simulink model "Microgrid"  (R2022b)
settings: Solver=ode45  StartTime=0.0  StopTime=0.5  RelTol=1e-3  EnableMultiTasking=on
model workspace (MAT data in the model file):
  AFPV = 1
  AFW = 1
  DG = 1
  pvc = 1
  wf1 = 1
undefined symbols (not defined in the file): BMSS1, D1, Delta, Ion, Lithium, R
libraries: spsDiodeLib x10, spsVoltageMeasurementLib x8, spsThreePhaseVIMeasurementLib x7, spsSeriesRLCBranchLib x7, fuzblock x6, spsMosfetLib x3, powerlib_extras x3, spsBreakerLib x2, spsThreePhaseParallelRLCLoadLib x2, spsThreePhaseBreakerLib x2, spsPWMGenerator2LevelLib x2, spsBatteryLib x1
(part 2 of 2)

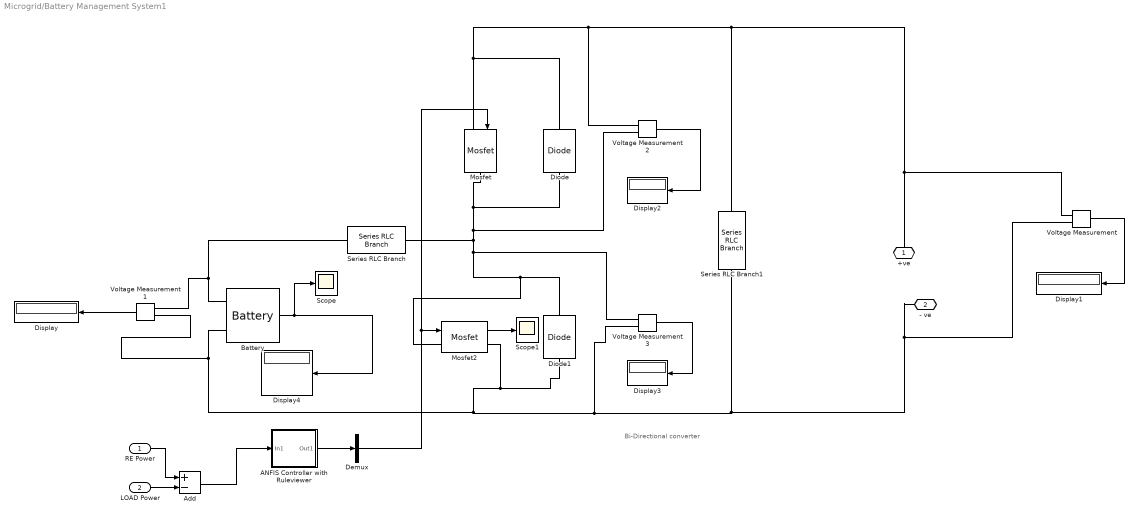
== system Microgrid/Battery Management System1 ==
  note: Bi-Directional converter
  RE Power : Inport
  LOAD Power : Inport  Port=2
  ANFIS Controller with Ruleviewer : Subsystem  AncestorBlock=|  mask(Fuzzy Inference System){fismatrix=[BMSS1], Ts=0.01}
      | fuzblock/Fuzzy Logic 
      | Controller 
      | with Ruleviewer
      mask prompts: fismatrix "fuzzy:dialogs:flcWithRuleViewerMaskPrompt_paramFIS"; Ts "fuzzy:dialogs:flcWithRuleViewerMaskPrompt_paramRate"
      mask help: fuzzy:dialogs:flcWithRuleViewerMask_description
      mask init:
      | fuzzy.internal.utility.errorIfType2FIS(fismatrix)
      settings: LibrarySourceBlock=|
      | fuzblock/Fuzzy Logic
      | Controller
      | with Ruleviewer
      mask Help: helpview(fullfile(docroot,'toolbox','fuzzy','fuzzy.map'), 'fuzviewerblock');
      mask DialogControl DescGroupVar Prompt: Fuzzy Inference System
      mask DialogControl fismatrix Prompt: FIS structure:
      mask DialogControl Ts Prompt: Refresh rate (s):
      mask Display: plot(0, -0.3, 6, -0.3, 0, 1.2, 6, 1.2, [0 6], [0 0], [1 2 3],[0 1 0],[2 3 4],[0 1 0],[3 4 5],[0 1 0])
  Add : Sum  Inputs=+-
  Battery : spsBatteryLib/Battery  BatType=Lithium-Ion  ShowTempParam=off  ThermalPreset=no  ShowAgeParam=off  NomV=200  NomQ=50  SOC=50  Batt_Tr=0.1  PresetModel=on  MaxQ=50  MinV=150  FullV=232.7974  Dis_rate=21.7391  R=0.04  Normal_OP=45.2174  expZone="[216.0772      2.456522]"  current=[5 10 15]  Units=Time  Tci=20  NomT=20  T2=-30  MaxQ2=4.8  FullV2=7.1  Normal_OP2=5.655  expZone2="[6.58           1]"  Rca=0.6  ti=2000  Dp=0  Neq0=0  Tsim=1e6  Ta1=25  Qeol=5.4*0.9  Reol=0.013333*1.2  Char_age=[2.3478, 3]  Dis_age=[2.3478, 10]  N1=1500  N2=10500  N3=1000  N4=1400  Ta2=45  N5=950
      settings: LibrarySourceBlock=electricdrivelib/Extra Sources/Battery
  Demux : Demux  Outputs=1
  Diode : spsDiodeLib/Diode  Ron=0.001  Lon=0  Vf=0.8  IC=0  UseSnubber=0  Rs=500  Cs=250e-9  Measurements=off
  Diode1 : spsDiodeLib/Diode  Ron=0.001  Lon=0  Vf=0.8  IC=0  UseSnubber=0  Rs=500  Cs=250e-9  Measurements=off
  Display{,1..4} (5 alike) : Display
  Mosfet : spsMosfetLib/Mosfet  Ron=0.1  Lon=0  Rd=0.01  Vfd=0  IC=0  Rs=1e5  Cs=inf  Measurements=off
  Mosfet2 : spsMosfetLib/Mosfet  Ron=0.1  Lon=0  Rd=0.01  Vfd=0  IC=0  Rs=1e5  Cs=inf  Measurements=on
  Scope : Scope
  Scope1 : Scope
  Series RLC Branch : spsSeriesRLCBranchLib/Series RLC Branch  LConnTagsString=__new0  RConnTagsString=__new0  BranchType=L  Resistance=1  Inductance=1e-3  SetiL0=off  InitialCurrent=0  Capacitance=1e-6  Setx0=off  InitialVoltage=0  Measurements=None
  Series RLC Branch1 : spsSeriesRLCBranchLib/Series RLC Branch  LConnTagsString=__new0  RConnTagsString=__new0  BranchType=RC  Resistance=1  Inductance=1e-3  SetiL0=off  InitialCurrent=0  Capacitance=1e-6  Setx0=off  InitialVoltage=0  Measurements=None
  Voltage Measurement{,1..3} (4 alike) : spsVoltageMeasurementLib/Voltage Measurement  PhasorSimulation=off  OutputType=Complex  PSBequivalent=0
  +ve : PMIOPort  Side=Right
  - ve : PMIOPort  Port=2  Side=Right
  wires:
  Voltage Measurement3/1 -> Display3/1
  Voltage Measurement2/1 -> Display2/1
  Voltage Measurement1/1 -> Display/1
  Voltage Measurement/1 -> Display1/1
  Battery/1 -> Scope/1, Display4/1
  ANFIS Controller with Ruleviewer/1(Out1) -> Demux/1
  Demux/1 -> Mosfet/1, Mosfet2/1
  Add/1 -> ANFIS Controller with Ruleviewer/1(In1)
  RE Power/1 -> Add/1
  LOAD Power/1 -> Add/2
  Mosfet2/1 -> Scope1/1
  connections:
  Mosfet/RConn1 -- Diode/LConn1 -- Voltage Measurement2/LConn2 -- Series RLC Branch/RConn1 -- Voltage Measurement3/LConn1 -- Mosfet2/LConn1 -- Diode1/RConn1
  Voltage Measurement1/LConn1 -- Series RLC Branch/LConn1 -- Battery/LConn1
  Mosfet/LConn1 -- Diode/RConn1 -- Voltage Measurement2/LConn1 -- Series RLC Branch1/LConn1 -- Voltage Measurement/LConn1 -- +ve/RConn1
  Diode1/LConn1 -- Mosfet2/RConn1 -- Battery/LConn2 -- Voltage Measurement1/LConn2 -- Voltage Measurement3/LConn2 -- Series RLC Branch1/RConn1 -- Voltage Measurement/LConn2 -- - ve/RConn1

== system Microgrid/Fuzzy Logic Controller with Ruleviewer ==
  In1 : Inport
  Fuzzy Logic Controller : fuzblock/Fuzzy Logic  Controller  FIS='tipper.fis'  OutputSampleNumber=101  DataType=double  FuzzifiedInputs=off  RuleFiringStrengths=off  RuleOutputs=off  AggregatedOutputs=off  SimulateUsing=Interpreted execution  OutOfRangeInputValueMessage=warning  NoRuleFiredMessage=warning  EmptyOutputFuzzySetMessage=warning
  Scope3 : Scope
  Zero-Order Hold : ZeroOrderHold  SampleTime=Ts
  Out1 : Outport  InitialOutput=0  VectorParamsAs1DForOutWhenUnconnected=off
  wires:
  In1/1 -> Fuzzy Logic Controller/1, Zero-Order Hold/1
  Fuzzy Logic Controller/1 -> Out1/1
  Zero-Order Hold/1 -> Scope3/1

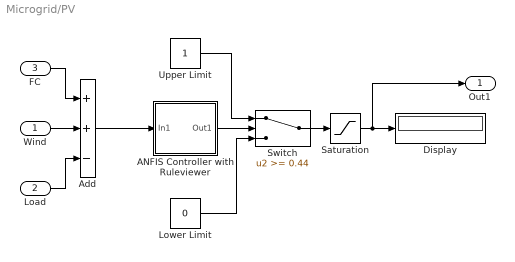
== system Microgrid/PV ==
  Wind : Inport
  Load : Inport  Port=2
  FC : Inport  Port=3
  ANFIS Controller with Ruleviewer : Subsystem  AncestorBlock=|  mask(Fuzzy Inference System){fismatrix=[pvc], Ts=0.01}
      | fuzblock/Fuzzy Logic 
      | Controller 
      | with Ruleviewer
      mask prompts: fismatrix "fuzzy:dialogs:flcWithRuleViewerMaskPrompt_paramFIS"; Ts "fuzzy:dialogs:flcWithRuleViewerMaskPrompt_paramRate"
      mask help: fuzzy:dialogs:flcWithRuleViewerMask_description
      mask init:
      | fuzzy.internal.utility.errorIfType2FIS(fismatrix)
      settings: LibrarySourceBlock=|
      | fuzblock/Fuzzy Logic
      | Controller
      | with Ruleviewer
      mask Help: helpview(fullfile(docroot,'toolbox','fuzzy','fuzzy.map'), 'fuzviewerblock');
      mask DialogControl DescGroupVar Prompt: Fuzzy Inference System
      mask DialogControl fismatrix Prompt: FIS structure:
      mask DialogControl Ts Prompt: Refresh rate (s):
      mask Display: plot(0, -0.3, 6, -0.3, 0, 1.2, 6, 1.2, [0 6], [0 0], [1 2 3],[0 1 0],[2 3 4],[0 1 0],[3 4 5],[0 1 0])
  Add : Sum  Inputs=++-
  Display : Display
  Lower Limit : Constant  Value=0
  Saturation : Saturate  UpperLimit=1  LowerLimit=0  LinearizeAsGain=off  ZeroCross=off
  Switch : Switch  Threshold=0.44  ZeroCross=off  SaturateOnIntegerOverflow=off  InputSameDT=off
  Upper Limit : Constant
  Out1 : Outport
  wires:
  Wind/1 -> Add/2
  Load/1 -> Add/3
  Add/1 -> ANFIS Controller with Ruleviewer/1(In1)
  Saturation/1 -> Out1/1, Display/1
  Switch/1 -> Saturation/1
  Upper Limit/1 -> Switch/1
  Lower Limit/1 -> Switch/3
  ANFIS Controller with Ruleviewer/1(Out1) -> Switch/2
  FC/1 -> Add/1

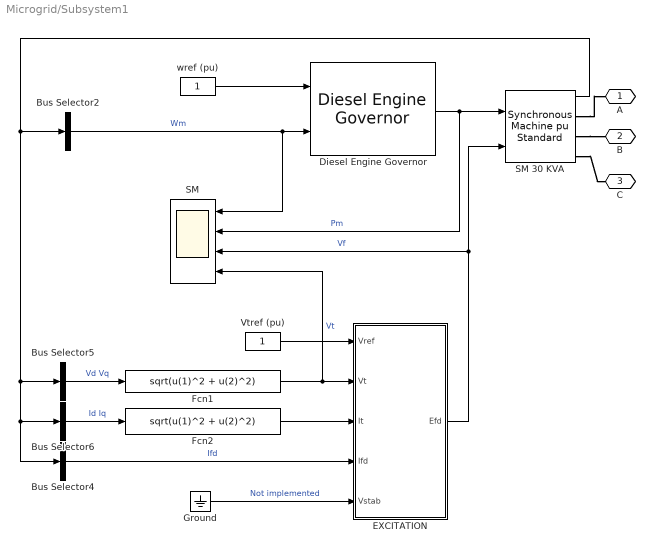
== system Microgrid/Subsystem1 ==
  Bus Selector2 : BusSelector  OutputSignals="Mechanical.Rotor speed  wm  (pu)"  OutputAsBus=on
  Bus Selector4 : BusSelector  OutputSignals="dq0 components.Field current  ifd (pu)"  OutputAsBus=on
  Bus Selector5 : BusSelector  OutputSignals="dq0 components.Stator voltage  vd (pu),dq0 components.Stator voltage  vq (pu)"  OutputAsBus=on
  Bus Selector6 : BusSelector  OutputSignals="dq0 components.Stator current  id (pu),dq0 components.Stator current  iq (pu)"  OutputAsBus=on
  Diesel Engine Governor : spsDieselMotorModel/Diesel Engine Governor  K=40  Tr=[0.01 0.02 0.2]  Ta=[0.25 0.009 0.0384]  Tlim=[0 1.1]  Td=0.024  Pm0=0
  EXCITATION : Subsystem  Variant=on  VariantControlMode=label  LabelModeActiveChoice=Variant1
      settings: AttributesFormatString=%<BlockChoice>
  Fcn1 : Fcn  Expr=sqrt(u(1)^2 + u(2)^2)
  Fcn2 : Fcn  Expr=sqrt(u(1)^2 + u(2)^2)
  Ground : Ground
  SM : Scope  NumInputPorts=4
  SM 30 KVA : spsSynchronousMachinepuStandardLib/Synchronous Machine pu Standard  PresetModel=No  MechanicalLoad=Mechanical power Pm  ShowDetailedParameters=on  RotorType=Salient-pole  Units=per unit standard parameters  MeasurementBus=off  NominalParameters="[ 30e3  350  50]"  Reactances1=[ 31 32 33 34 35 36 37 ]  Reactances2=[ 1.56, 0.296, 0.177, 1.06, 0.177, 0.052 ]  dAxisTimeConstants=Short-circuit  qAxisTimeConstants=Open-circuit  TimeConstants1=[]  TimeConstants2=[]  TimeConstants3=[]  TimeConstants4=[]  TimeConstants5=[ 3.7, 0.05, 0.05 ]  TimeConstants6=[ 8.0, 0.03, 0.3371, 0.0295 ]  TimeConstants7=[0.024 0.006 0.006]  TimeConstants8=[]  StatorResistance=0.0036  Mechanical="[ 1.07  0 2]"  PolePairs=2  InitialConditions=[0 0 0 0 0 0 0 0 1]  SetSaturation=off  Saturation=[0.211 0.418 1.0 1.25 1.72 3.35 ;0.25 0.50 1.0 1.1 1.2 1.4]  LoadFlowParameters=[1 0 0 0]  TsPowergui=0  TsBlock=-1  IterativeModel=Trapezoidal non iterative  IterativeDiscreteModel=Trapezoidal non iterative  BusType=PV  Pref=0  Qref=0  Qmin=-Inf  Qmax=Inf  PLF=0  QLF=0
  "Vtref (pu) " : Constant
  wref (pu) : Constant
  A : PMIOPort  Side=Right
  B : PMIOPort  Port=2  Side=Right
  C : PMIOPort  Port=3  Side=Right
  wires:
  Bus Selector6/1 -> Fcn2/1  "Id Iq"
  SM 30 KVA/1 -> Bus Selector2/1, Bus Selector5/1, Bus Selector6/1, Bus Selector4/1
  "Vtref (pu) "/1 -> EXCITATION/1(Vref)
  Bus Selector2/1 -> Diesel Engine Governor/2, SM/1  "Wm"
  EXCITATION/1(Efd) -> SM/3, SM 30 KVA/2  "Vf"
  Bus Selector4/1 -> EXCITATION/4(Ifd)  "Ifd"
  wref (pu)/1 -> Diesel Engine Governor/1
  Bus Selector5/1 -> Fcn1/1  "Vd Vq"
  Fcn1/1 -> SM/4, EXCITATION/2(Vt)  "Vt"
  Diesel Engine Governor/1 -> SM/2, SM 30 KVA/1  "Pm"
  Fcn2/1 -> EXCITATION/3(It)
  Ground/1 -> EXCITATION/5(Vstab)  "Not implemented"
  connections:
  SM 30 KVA/RConn1 -- A/RConn1
  SM 30 KVA/RConn3 -- C/RConn1
  SM 30 KVA/RConn2 -- B/RConn1

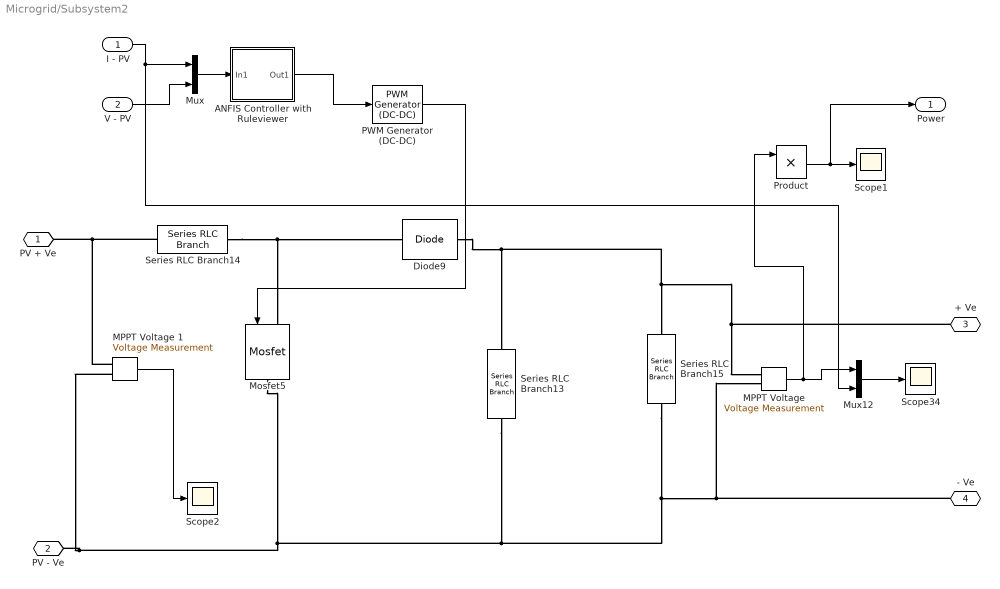
== system Microgrid/Subsystem2 ==
  I - PV : Inport
  V - PV : Inport  Port=2
  ANFIS Controller with Ruleviewer : Subsystem  AncestorBlock=|  mask(Fuzzy Inference System){fismatrix=[AFPV], Ts=0.01}
      | fuzblock/Fuzzy Logic 
      | Controller 
      | with Ruleviewer
      mask prompts: fismatrix "fuzzy:dialogs:flcWithRuleViewerMaskPrompt_paramFIS"; Ts "fuzzy:dialogs:flcWithRuleViewerMaskPrompt_paramRate"
      mask help: fuzzy:dialogs:flcWithRuleViewerMask_description
      mask init:
      | fuzzy.internal.utility.errorIfType2FIS(fismatrix)
      settings: LibrarySourceBlock=|
      | fuzblock/Fuzzy Logic
      | Controller
      | with Ruleviewer
      mask Help: helpview(fullfile(docroot,'toolbox','fuzzy','fuzzy.map'), 'fuzviewerblock');
      mask DialogControl DescGroupVar Prompt: Fuzzy Inference System
      mask DialogControl fismatrix Prompt: FIS structure:
      mask DialogControl Ts Prompt: Refresh rate (s):
      mask Display: plot(0, -0.3, 6, -0.3, 0, 1.2, 6, 1.2, [0 6], [0 0], [1 2 3],[0 1 0],[2 3 4],[0 1 0],[3 4 5],[0 1 0])
  Diode9 : spsDiodeLib/Diode  Ron=0.001  Lon=0  Vf=0.8  IC=0  UseSnubber=off  Rs=500  Cs=250e-9  Measurements=off
  "MPPT Voltage " : spsVoltageMeasurementLib/Voltage Measurement  PhasorSimulation=off  OutputType=Complex  PSBequivalent=0
  MPPT Voltage 1 : spsVoltageMeasurementLib/Voltage Measurement  PhasorSimulation=off  OutputType=Complex  PSBequivalent=0
  Mosfet5 : spsMosfetLib/Mosfet  Ron=0.1  Lon=0  Rd=0.01  Vfd=0  IC=0  Rs=1e5  Cs=inf  Measurements=off
  Mux : Mux  Inputs=2
  Mux12 : Mux  Inputs=2
  PWM Generator (DC-DC) : spsPWMGeneratorDCDCLib/PWM Generator (DC-DC)  Fsw=5000  Ts=0
  Product : Product
  Scope1 : Scope
  Scope2 : Scope
  Scope34 : Scope
  Series RLC Branch13 : spsSeriesRLCBranchLib/Series RLC Branch  LConnTagsString=__new0  RConnTagsString=__new0  BranchType=C  Resistance=1  Inductance=1e-3  SetiL0=off  InitialCurrent=0  Capacitance=550e-6  Setx0=off  InitialVoltage=0  Measurements=None
  Series RLC Branch14 : spsSeriesRLCBranchLib/Series RLC Branch  LConnTagsString=__new0  RConnTagsString=__new0  BranchType=L  Resistance=1  Inductance=0.05e-2  SetiL0=off  InitialCurrent=0  Capacitance=1e-6  Setx0=off  InitialVoltage=0  Measurements=None
  Series RLC Branch15 : spsSeriesRLCBranchLib/Series RLC Branch  LConnTagsString=__new0  RConnTagsString=__new0  BranchType=R  Resistance=20  Inductance=1e-3  SetiL0=off  InitialCurrent=0  Capacitance=1e-6  Setx0=off  InitialVoltage=0  Measurements=None
  PV + Ve : PMIOPort  Side=Left
  PV - Ve : PMIOPort  Port=2  Side=Left
  + Ve : PMIOPort  Port=3  Side=Right
  - Ve : PMIOPort  Port=4  Side=Right
  Power : Outport
  wires:
  MPPT Voltage 1/1 -> Scope2/1
  Mux12/1 -> Scope34/1
  "MPPT Voltage "/1 -> Product/1, Mux12/1
  I - PV/1 -> Mux/1, Mux12/2
  ANFIS Controller with Ruleviewer/1(Out1) -> PWM Generator (DC-DC)/1
  PWM Generator (DC-DC)/1 -> Mosfet5/1
  V - PV/1 -> Mux/2
  Product/1 -> Power/1, Scope1/1
  Mux/1 -> ANFIS Controller with Ruleviewer/1(In1)
  connections:
  MPPT Voltage 1/LConn1 -- Series RLC Branch14/LConn1 -- PV + Ve/RConn1
  MPPT Voltage 1/LConn2 -- PV - Ve/RConn1 -- Series RLC Branch13/RConn1 -- - Ve/RConn1 -- "MPPT Voltage "/LConn2 -- Series RLC Branch15/RConn1 -- Mosfet5/RConn1
  + Ve/RConn1 -- Series RLC Branch13/LConn1 -- Diode9/RConn1 -- Series RLC Branch15/LConn1 -- "MPPT Voltage "/LConn1
  Series RLC Branch14/RConn1 -- Diode9/LConn1 -- Mosfet5/LConn1

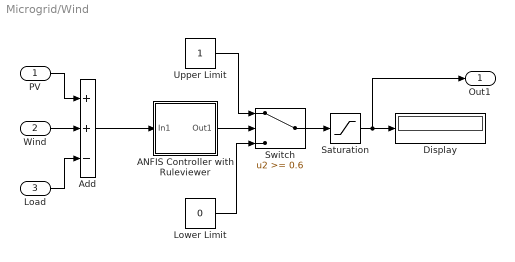
== system Microgrid/Wind ==
  PV : Inport
  Wind : Inport  Port=2
  Load : Inport  Port=3
  ANFIS Controller with Ruleviewer : Subsystem  AncestorBlock=|  mask(Fuzzy Inference System){fismatrix=[wf1], Ts=0.01}
      | fuzblock/Fuzzy Logic 
      | Controller 
      | with Ruleviewer
      mask prompts: fismatrix "fuzzy:dialogs:flcWithRuleViewerMaskPrompt_paramFIS"; Ts "fuzzy:dialogs:flcWithRuleViewerMaskPrompt_paramRate"
      mask help: fuzzy:dialogs:flcWithRuleViewerMask_description
      mask init:
      | fuzzy.internal.utility.errorIfType2FIS(fismatrix)
      settings: LibrarySourceBlock=|
      | fuzblock/Fuzzy Logic
      | Controller
      | with Ruleviewer
      mask Help: helpview(fullfile(docroot,'toolbox','fuzzy','fuzzy.map'), 'fuzviewerblock');
      mask DialogControl DescGroupVar Prompt: Fuzzy Inference System
      mask DialogControl fismatrix Prompt: FIS structure:
      mask DialogControl Ts Prompt: Refresh rate (s):
      mask Display: plot(0, -0.3, 6, -0.3, 0, 1.2, 6, 1.2, [0 6], [0 0], [1 2 3],[0 1 0],[2 3 4],[0 1 0],[3 4 5],[0 1 0])
  Add : Sum  Inputs=++-
  Display : Display
  Lower Limit : Constant  Value=0
  Saturation : Saturate  UpperLimit=1  LowerLimit=0  LinearizeAsGain=off  ZeroCross=off
  Switch : Switch  Threshold=0.6  ZeroCross=off  SaturateOnIntegerOverflow=off  InputSameDT=off
  Upper Limit : Constant
  Out1 : Outport
  wires:
  ANFIS Controller with Ruleviewer/1(Out1) -> Switch/2
  Lower Limit/1 -> Switch/3
  Upper Limit/1 -> Switch/1
  Switch/1 -> Saturation/1
  Saturation/1 -> Display/1, Out1/1
  Add/1 -> ANFIS Controller with Ruleviewer/1(In1)
  PV/1 -> Add/1
  Load/1 -> Add/3
  Wind/1 -> Add/2

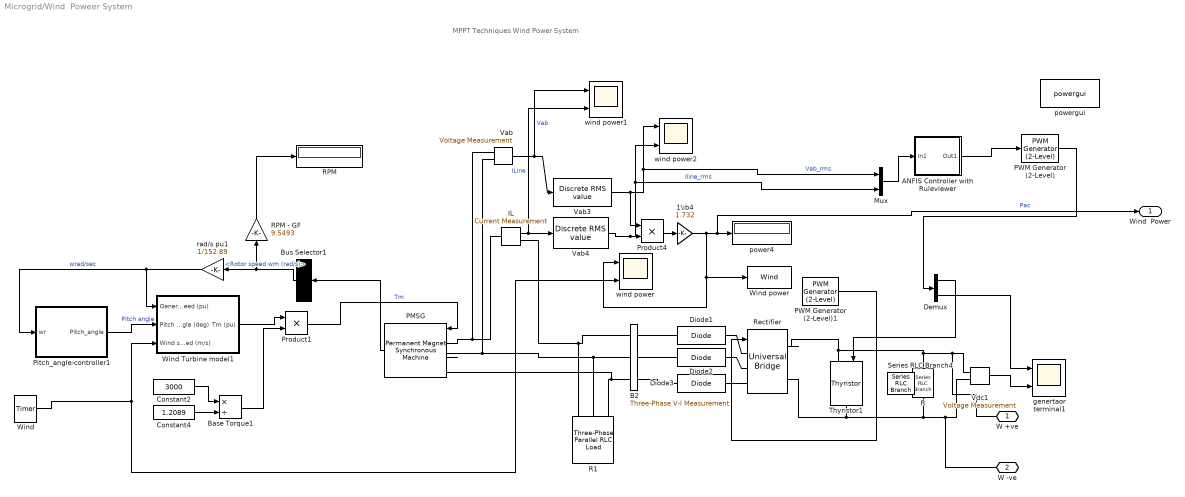
== system Microgrid/Wind  Poweer System ==
  note: MPPT Techniques Wind Power System
  1\ib4 : Gain  Gain=1.732  SaturateOnIntegerOverflow=on  OutDataTypeStr=Inherit: Same as input  ParamDataTypeStr=Inherit: Same as input
  ANFIS Controller with Ruleviewer : Subsystem  AncestorBlock=|  mask(Fuzzy Inference System){fismatrix=[AFW], Ts=0.01}
      | fuzblock/Fuzzy Logic 
      | Controller 
      | with Ruleviewer
      mask prompts: fismatrix "fuzzy:dialogs:flcWithRuleViewerMaskPrompt_paramFIS"; Ts "fuzzy:dialogs:flcWithRuleViewerMaskPrompt_paramRate"
      mask help: fuzzy:dialogs:flcWithRuleViewerMask_description
      mask init:
      | fuzzy.internal.utility.errorIfType2FIS(fismatrix)
      settings: LibrarySourceBlock=|
      | fuzblock/Fuzzy Logic
      | Controller
      | with Ruleviewer
      mask Help: helpview(fullfile(docroot,'toolbox','fuzzy','fuzzy.map'), 'fuzviewerblock');
      mask DialogControl DescGroupVar Prompt: Fuzzy Inference System
      mask DialogControl fismatrix Prompt: FIS structure:
      mask DialogControl Ts Prompt: Refresh rate (s):
      mask Display: plot(0, -0.3, 6, -0.3, 0, 1.2, 6, 1.2, [0 6], [0 0], [1 2 3],[0 1 0],[2 3 4],[0 1 0],[3 4 5],[0 1 0])
  "B2 " : spsThreePhaseVIMeasurementLib/Three-Phase V-I Measurement  VoltageMeasurement=no  SetLabelV=on  LabelV=Vabc_B2  Vpu=off  VpuLL=off  CurrentMeasurement=no  SetLabelI=on  LabelI=Iabc_B2  Ipu=off  Pbase=100e6  Vbase=500e3  OutputType=Magnitude  PhasorSimulation=off  PSBequivalent=0
  Base Torque1 : Product  Inputs=*/  RndMeth=Zero
  Bus Selector1 : BusSelector  OutputSignals=Rotor speed wm (rad/s)
  Constant2 : Constant  Value=3000
  Constant4 : Constant  Value=1.2089
  Demux : Demux  Outputs=2
  Diode1 : spsDiodeLib/Diode  Ron=0.001  Lon=0  Vf=0.8  IC=0  UseSnubber=off  Rs=500  Cs=250e-9  Measurements=off
  Diode2 : spsDiodeLib/Diode  Ron=0.001  Lon=0  Vf=0.8  IC=0  UseSnubber=off  Rs=500  Cs=250e-9  Measurements=off
  Diode3 : spsDiodeLib/Diode  Ron=0.001  Lon=0  Vf=0.8  IC=0  UseSnubber=off  Rs=500  Cs=250e-9  Measurements=off
  IL : spsCurrentMeasurementLib/Current Measurement  PhasorSimulation=off  OutputType=Complex  PSBequivalent=0
  Mux : Mux  Inputs=2
  PMSG : spsPermanentMagnetSynchronousMachineLib/Permanent Magnet Synchronous Machine  NbPhases=3  FluxDistribution=Sinusoidal  RotorType=Round  MechanicalLoad=Torque Tm  PresetModel=No  ShowDetailedParameters=on  MeasurementBus=off  Resistance=0.0918  Inductance=8.5e-3  dqInductances=[0.0082 0.0082]  La=0.000975  MachineConstant=Flux linkage established by magnets (V.s)  Flux=0.1688  VoltageCst=122.4677  TorqueCst=1.0128  Flat=120  Mechanical=[0.003945 0.0004924 4 0]  PolePairs=4  InitialConditions=[0,0, 0,0]  InitialConditions5ph=[0 0 0 0 0 0]  RefAngle=90 degrees behind phase A axis (modified Park)  IterativeDiscreteModel=Trapezoidal non iterative  TsBlock=-1  TsPowergui=0
  PWM Generator (2-Level) : spsPWMGenerator2LevelLib/PWM Generator (2-Level)  ModulatorType=Single-phase half-bridge (2 pulses)  ModulatorMode=Unsynchronized  Fc=3000  Pc=90  nF=27  MinMax="[ -1  1 ]"  SamplingTechnique=Natural  ModulatingSignals=off  m=0.8  Freq=60  Phase=0  Ts=0  ShowCarrierOutport=off
  PWM Generator (2-Level)1 : spsPWMGenerator2LevelLib/PWM Generator (2-Level)  ModulatorType=Three-phase bridge (6 pulses)  ModulatorMode=Unsynchronized  Fc=27*60  Pc=90  nF=27  MinMax="[ -1  1 ]"  SamplingTechnique=Natural  ModulatingSignals=on  m=0.7  Freq=50  Phase=0  Ts=0  ShowCarrierOutport=off
  Pitch_angle-controller1 : Subsystem
  Product1 : Product  RndMeth=Zero
  Product4 : Product  RndMeth=Zero
  R : spsSeriesRLCBranchLib/Series RLC Branch  LConnTagsString=__new0  RConnTagsString=__new0  BranchType=R  Resistance=20  Inductance=1e-3  SetiL0=off  InitialCurrent=0  Capacitance=1e-6  Setx0=off  InitialVoltage=0  Measurements=None
  "R1 " : spsThreePhaseParallelRLCLoadLib/Three-Phase Parallel RLC Load  LConnTagsString=A|B|C  Configuration=Y (grounded)  NominalVoltage=220  Vabc=[1e3 1e3 1e3]  Vabcp=[1e3 1e3 1e3]  NominalFrequency=50  UnbalancedPower=off  ActivePower=24000  InductivePower=0  CapacitivePower=0  Pabc=[9e3 9e3 9e3]  QLabc=[100 90 110]  QCabc=[100 90 110]  Pabcp=[10e3 9e3 11e3]  QLabcp=[100 90 110]  QCabcp=[100 90 110]  Measurements=None  LoadType=constant Z
  "RPM " : Display
  RPM - GF : Gain  Gain=9.5493  SaturateOnIntegerOverflow=on  OutDataTypeStr=Inherit: Same as input  ParamDataTypeStr=Inherit: Same as input
  Rectifier : spsUniversalBridgeLib/Universal Bridge  Arms=3  SnubberResistance=100  SnubberCapacitance=0.1e-6  Device=IGBT / Diodes  Ron=1e-3  Lon=0  ForwardVoltages="[  100  100  ]"  ForwardVoltage=.8  GTOparameters=[ 10e-6 , 20e-6 ]  IGBTparameters=[ 1e-6 , 2e-6 ]  Measurements=Device currents  Measurements_2=None  converterType=Rectifier
      settings: AttributesFormatString=\n
  Series RLC Branch4 : spsSeriesRLCBranchLib/Series RLC Branch  LConnTagsString=__new0  RConnTagsString=__new0  BranchType=C  Resistance=R  Inductance=1e-3  SetiL0=off  InitialCurrent=0  Capacitance=470e-5  Setx0=off  InitialVoltage=0  Measurements=Branch voltage and current
  Thyristor1 : spsThyristorLib/Thyristor  Ron=0.001  Lon=0  Vf=220  IC=0  Rs=500  Cs=250e-9  Measurements=off
  Vab : spsVoltageMeasurementLib/Voltage Measurement  PhasorSimulation=off  OutputType=Complex  PSBequivalent=0
  Vab3 : powerlib_extras/Discrete Measurements/Discrete  RMS value  Freq=50  Mag_Init=0  Ts=20e-6
  Vab4 : powerlib_extras/Discrete Measurements/Discrete  RMS value  Freq=50  Mag_Init=0  Ts=20e-6
  Vdc1 : spsVoltageMeasurementLib/Voltage Measurement  Tag=PoWeRsYsTeMmEaSuReMeNt  PhasorSimulation=off  OutputType=Magnitude  PSBequivalent=0
  "Wind " : powerlib_extras/Control  Blocks/Timer  t=[0 0.05 0.1 0.15 0.2 ]  e=[5 7 11 12 12]
  Wind Turbine model1 : Subsystem  AncestorBlock=DRlib/Wind Generation/Wind Turbine  DialogController=POWERSYS.PowerSysDialog  mask(Wind Turbine){Pnom=20000, Pelec_base=20000/0.9, wind_base=12, P_wind_base=0.8, speed_nom=1, pitch_angle=0, DisplayTurbChar=off, c1_c6=[0.51763          116          0.4            5           21     0.006795], cp_nom=0.48, lambda_nom=8.1}
      mask prompts: Pnom "Nominal mechanical output power (W):"; Pelec_base "Base power of the electrical generator (VA):"; wind_base "Base wind speed (m/s):"; P_wind_base "Maximum power at base wind speed (pu of nominal mechanical power):"; speed_nom "Base rotational speed (p.u. of base generator speed):"; pitch_angle "Pitch angle beta to display wind-turbine power characteristics (beta >=0)  (deg):"; DisplayTurbChar "Display wind turbine power characteristics"
      mask help:
      | This block implements a variable pitch wind turbine model. The performance coefficient Cp of the turbine is the mechanical output power of the turbine divided by wind power and a function of wind speed, rotational speed, and pitch angle (beta). Cp reaches its maximum value at zero beta. Select the wind-turbine power characteristics display to plot the turbine characteristics at the specified pitch angle.
      |
      | The first input is the generator speed in per unit of the generator base speed. For a synchronous or asynchronous generator, the base speed is the synchronous speed. For a permanent-magnet generator, the base speed is defined as the speed producing nominal voltage at  no load. The second input is the blade pitch angle (beta) in degrees. The third input is the wind speed in m/s.
      |
      | The output is the torque applied to the generator shaft in per unit of the generator ratings.
      |
      | The turbine inertia must be added to the generator inertia.
      mask init:
      | %Wind turbine typical characteristic data
      | %c2=116;c3=0.4;c4=5;c5=21;
      | %Computation of c1 and c6 for lambda_nom et cpmax
      | %lambda_nom=8.1;
      | %cp_max=0.48;
      | %cp_nom=cp_max;
      | 
      | %lambda_i_nom=1/(1/lambda_nom-0.035);
      | %k_nom=-(c2*c5/lambda_i_nom-c4*c5-c2)*exp(-c5/lambda_i_nom)/lambda_nom^2;
      | %c1=cp_max/((c2/lambda_i_nom-c4)*exp(-c5/lambda_i_nom)+k_nom*lambda_nom);
      | %c6=k_nom*c1;
      | power_initmask();
      settings: LibrarySourceBlock=DRlib/Wind Generation/Wind Turbine
      mask Help: web(psbhelp);
      mask Callback Pnom:
      | ParVisible={'on','on','on','on','on','on','on','off','off','off',};
      | set_param(gcb,'MaskVisibilities',ParVisible);
      | c1_c6=str2num(get_param(gcb,'c1_c6'));
      | c1=c1_c6(1);c2=c1_c6(2);c3=c1_c6(3);c4=c1_c6(4);c5=c1_c6(5);c6=c1_c6(6);
      mask Callback DisplayTurbChar:
      | DisplayTurbChar=get_param(gcb,'DisplayTurbChar');
      | 
      | if strcmp(DisplayTurbChar,'on')
      |     fig_num=figure;
      | 	clf(fig_num);
      | 	[speed_nom,wind_base,P_wind_base,pitch_angle]=getSPSmaskvalues(gcb,{'speed_nom','wind_base','P_wind_base','pitch_angle'});
      | 	[c1_c6,lambda_nom,cp_nom]=getSPSmaskvalues(gcb,{'c1_c6','lambda_nom','cp_nom'});
      | 	c1=c1_c6(1);c2=c1_c6(2);c3=c1_c6(3);c4=c1_c6(4);c5=c1_c6(5);c6=c1_c6(6);
      | 
      | 	%Wind turbine typical characteristic data
      |     %c2=116;c3=0.4;c4=5;c5=21;
      |     %Computation of c1 and c6 for lambda_nom et cpmax
      |     %lambda_nom=8.1;
      |     %cp_max=0.48;
      |     %cp_nom=cp_max;
      | 
      |     %lambda_i_nom=1/(1/lambda_nom-0.035);
      |     %k_nom=-(c2*c5/lambda_i_nom-c4*c5-c2)*exp(-c5/lambda_i_nom)/lambda_nom^2;
      |     %c1=cp_max/((c2/lambda_i_nom-c4)*exp(-c5/lambda_i_nom)+k_nom*lambda_nom);
      |     %c6=k_nom*c1;
      | 
      | 	wr_elec_pu=1e-3:0.01:1.5;;
      |     wr_mec_pu=wr_elec_pu/speed_nom;
      |     wind_max=ceil((1.2/P_wind_base)^(1/3)*wind_base);
      |     wind_min=round(((0.1)/P_wind_base)^(1/3)*wind_base);
      |     wind1=wind_min:(wind_base-wind_min)/5:wind_base;
      |     wind2=wind_base+(wind_base-wind_min)/5:(wind_base-wind_min)/5:wind_max;
      |     wind_pu=[wind1 wind2]/wind_base;
      | 
      |     for k=1:length(wind_pu)
      |         for i=1:length(wr_mec_pu);
      |             lambda_pu=wr_mec_pu(i)/wind_pu(k);
      |             lambda=lambda_pu*lambda_nom;
      |             lambda_i=1/(1/(lambda+0.08*pitch_angle)-0.035/(pitch_angle^3+1));
      |             cp=c1*(c2/lambda_i-c3*pitch_angle-c4)*exp(-c5/lambda_i)+c6*lambda;
      |             cp_pu=cp/cp_nom;
      |             Pwind_pu(k,i)=wind_pu(k)^3*cp_pu*P_wind_base;
      |         end
      |     end
      |     for k=1:length(wind_pu)
      |         plot(wr_elec_pu,Pwind_pu(k,:))
      |         hold on
      |     end
      | 
      |     plot([speed_nom,speed_nom,0],[0,P_wind_base,P_wind_base],'r--')
      |     text(speed_nom+0.01,0+0.05,sprintf('%0.4g pu',speed_nom))
      |     text(0.01,P_wind_base+0.05,sprintf('Max. power at base wind speed (%0.4g m/s) and beta = 0 deg',wind_base))
      |     for i=1:length(wind_pu),
      |         p_max(i)=max(Pwind_pu(i,:));
      |         speed(i)=wr_elec_pu(find(Pwind_pu(i,:)==p_max(i)));
      |         text(speed(i),p_max(i),sprintf('%0.4g m/s',wind_pu(i)*wind_base))
      |     end
      |     plot([0 max(wr_elec_pu)],[0 0],'--')
      | 
      |     xlabel('Turbine speed (pu of nominal generator speed)')
      |     ylabel('Turbine output power (pu of nominal mechanical power)')
      |     title(sprintf('Turbine Power Characteristics (Pitch angle beta = %0.4g deg)',pitch_angle))
      |     axis([0 max(wr_elec_pu) min(Pwind_pu(1,:)) max(P_wind_base+0.1,max(wind_pu)^3*P_wind_base+0.1)])
      |     set_param(gcb,'DisplayTurbChar','off')
      | end
      mask Display: disp('');
  Wind power : ToWorkspace  VariableName=Wind  SaveFormat=Timeseries  SampleTime=-1
  genertaor terminal1 : Scope  NumInputPorts=2
  power4 : Display
      settings: SampleTime=1e-3
  powergui : spspowerguiLib/powergui  Priority=1  SimulationMode=Continuous  SampleTime=50e-6  frequency=60  Iterations=50  frequencyindice=0  Pbase=100e6  ErrMax=1e-4  UnitsV=kV  UnitsW=MW  buscounter=0  FunctionMessages=off  echomessages=off  EnableUseOfTLC=off  CurrentSourceSwitches=off  DisableSnubberDevices=off  DisableRonSwitches=off  DisableVfSwitches=off  DisplayEquations=off  AutomaticDiscreteSolvers=off  SolverType=Tustin/Backward Euler (TBE)  Interpol=off  ExternalGateDelay=off  methode=off  Ts=100  x0status=blocks  SPID=on  SwTol=0  HookPort=off  NonlinearTolerance=1e-4  nMaxIteration=100  ContinueOnMaxIteration=off  RestoreLinks=warning  ResistiveCurrentMeasurement=off  Frange=[0:2:500]  Ylog=off  Xlog=on  ShowGrid=off  save=off  variable=ZData  structure=0  ZoomFFT=off  StartTime=0.0  cycles=1  DisplayStyle=1  fundamental=60  FreqAxis=off  MaxFrequency=1000  frequencyindicesteady=1  RmsSteady=1  display=off
  rad/s pu1 : Gain  Gain=1/152.89  SaturateOnIntegerOverflow=on  OutDataTypeStr=Inherit: Same as input  ParamDataTypeStr=Inherit: Same as input
  wind power : Scope  NumInputPorts=2
  wind power1 : Scope  NumInputPorts=2
  wind power2 : Scope  NumInputPorts=2
  W +ve : PMIOPort  Side=Right
  W -ve : PMIOPort  Port=2  Side=Right
  Wind  Power : Outport
  wires:
  PMSG/1 -> Bus Selector1/1
  rad/s pu1/1 -> Pitch_angle-controller1/1(wr), Wind Turbine model1/1(Generator speed (pu))  "wrad/sec"
  Product1/1 -> PMSG/1  "Tm"
  Vab3/1 -> Product4/1, Mux/1, wind power2/1  "Vab_rms"
  Product4/1 -> 1\ib4/1
  Bus Selector1/1 -> RPM - GF/1, rad/s pu1/1  "<Rotor speed wm (rad/s)>"
  1\ib4/1 -> Wind  Power/1, power4/1, Wind power/1, wind power/1  "Pac"
  Vab/1 -> wind power1/1, Vab3/1  "Vab"
  Vdc1/1 -> genertaor terminal1/2
  "Wind "/1 -> Wind Turbine model1/3(Wind speed (m/s)), wind power/2
  Vab4/1 -> Mux/2, wind power2/2, Product4/2  "Iline_rms"
  Pitch_angle-controller1/1(Pitch_angle) -> Wind Turbine model1/2(Pitch angle (deg))  "Pitch angle"
  Constant2/1 -> Base Torque1/1
  Base Torque1/1 -> Product1/2
  IL/1 -> wind power1/2, Vab4/1  "ILine"
  Wind Turbine model1/1(Tm (pu)) -> Product1/1
  RPM - GF/1 -> "RPM "/1
  Constant4/1 -> Base Torque1/2
  Mux/1 -> ANFIS Controller with Ruleviewer/1(In1)
  ANFIS Controller with Ruleviewer/1(Out1) -> PWM Generator (2-Level)/1
  PWM Generator (2-Level)/1 -> Demux/1
  Demux/1 -> Thyristor1/1
  PWM Generator (2-Level)1/1 -> Rectifier/1
  Demux/2 -> genertaor terminal1/1
  connections:
  W +ve/RConn1 -- Vdc1/LConn1 -- R/LConn1 -- Rectifier/RConn1 -- Thyristor1/LConn1
  Rectifier/RConn2 -- Vdc1/LConn2 -- W -ve/RConn1 -- R/RConn1 -- Thyristor1/RConn1
  Diode2/RConn1 -- Rectifier/LConn2
  IL/RConn1 -- "B2 "/LConn1 -- "R1 "/LConn1
  PMSG/LConn2 -- Vab/LConn2 -- "B2 "/LConn2 -- "R1 "/LConn2
  "B2 "/RConn3 -- Diode3/LConn1
  PMSG/LConn1 -- Vab/LConn1 -- IL/LConn1
  "B2 "/LConn3 -- PMSG/LConn3 -- "R1 "/LConn3
  Diode1/RConn1 -- Rectifier/LConn1
  Diode1/LConn1 -- "B2 "/RConn1
  Diode3/RConn1 -- Rectifier/LConn3
  Diode2/LConn1 -- "B2 "/RConn2

== system Microgrid/Battery Management System1/ANFIS Controller with Ruleviewer ==
  In1 : Inport
  Fuzzy Logic Controller : fuzblock/Fuzzy Logic  Controller  FIS='tipper.fis'  OutputSampleNumber=101  DataType=double  FuzzifiedInputs=off  RuleFiringStrengths=off  RuleOutputs=off  AggregatedOutputs=off  SimulateUsing=Interpreted execution  OutOfRangeInputValueMessage=warning  NoRuleFiredMessage=warning  EmptyOutputFuzzySetMessage=warning
  Scope3 : Scope
  Zero-Order Hold : ZeroOrderHold  SampleTime=Ts
  Out1 : Outport  InitialOutput=0  VectorParamsAs1DForOutWhenUnconnected=off
  wires:
  In1/1 -> Fuzzy Logic Controller/1, Zero-Order Hold/1
  Fuzzy Logic Controller/1 -> Out1/1
  Zero-Order Hold/1 -> Scope3/1

== system Microgrid/PV/ANFIS Controller with Ruleviewer ==
  In1 : Inport
  Fuzzy Logic Controller : fuzblock/Fuzzy Logic  Controller  FIS='tipper.fis'  OutputSampleNumber=101  DataType=double  FuzzifiedInputs=off  RuleFiringStrengths=off  RuleOutputs=off  AggregatedOutputs=off  SimulateUsing=Interpreted execution  OutOfRangeInputValueMessage=warning  NoRuleFiredMessage=warning  EmptyOutputFuzzySetMessage=warning
  Scope3 : Scope
  Zero-Order Hold : ZeroOrderHold  SampleTime=Ts
  Out1 : Outport  InitialOutput=0  VectorParamsAs1DForOutWhenUnconnected=off
  wires:
  In1/1 -> Fuzzy Logic Controller/1, Zero-Order Hold/1
  Fuzzy Logic Controller/1 -> Out1/1
  Zero-Order Hold/1 -> Scope3/1

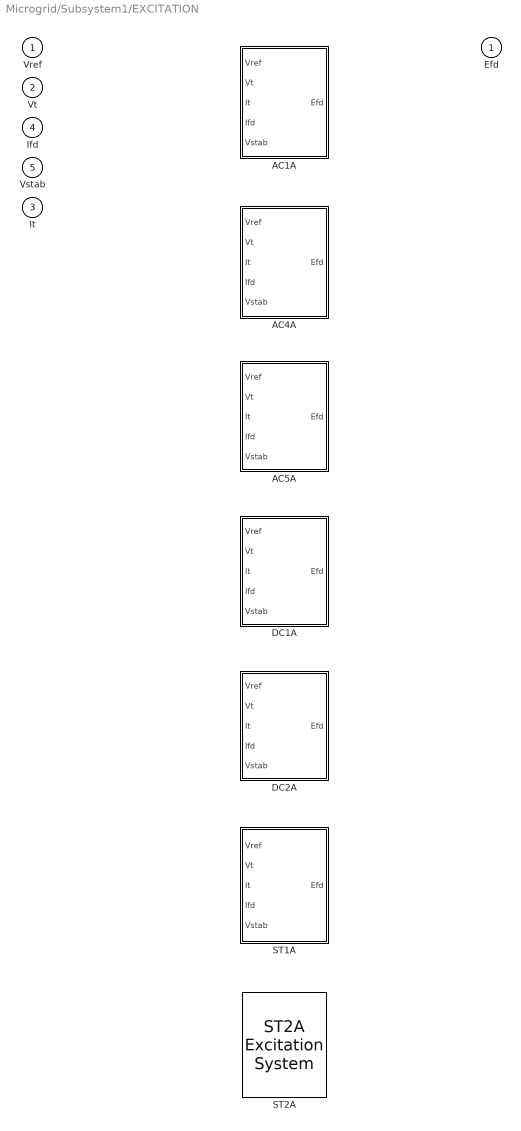
== system Microgrid/Subsystem1/EXCITATION ==
  Vref : Inport
  Vt : Inport  Port=2
  It : Inport  Port=3
  Ifd : Inport  Port=4
  Vstab : Inport  Port=5
  AC1A : Subsystem  VariantControl=Variant1
  AC4A : Subsystem  VariantControl=Variant2
  AC5A : Subsystem  VariantControl=Variant3
  DC1A : Subsystem  VariantControl=Variant4
  DC2A : Subsystem  VariantControl=Variant5
  ST1A : Subsystem  VariantControl=Variant6
  ST2A : spsST2AExcitationSystemLib/ST2A Excitation System  VariantControl=Variant7  Tr=20e-3  KaTa=[120 0.15]  VRminmax=[0 1.0]  KfTf=[0.05 1.0]  KeTe=[1.0 0.5]  KI=8.0  Kp=4.88  Xd=1.56  Kc=1.82  v0=[1,1.42734]  I0=0.2739  TsBlock=-2
      settings: LibrarySourceBlock=|
      | sps_lib/Electrical Machines/Synchronous Machine Control/ST2A
      | Excitation System
  Efd : Outport

== system Microgrid/Subsystem2/ANFIS Controller with Ruleviewer ==
  In1 : Inport
  Fuzzy Logic Controller : fuzblock/Fuzzy Logic  Controller  FIS='tipper.fis'  OutputSampleNumber=101  DataType=double  FuzzifiedInputs=off  RuleFiringStrengths=off  RuleOutputs=off  AggregatedOutputs=off  SimulateUsing=Interpreted execution  OutOfRangeInputValueMessage=warning  NoRuleFiredMessage=warning  EmptyOutputFuzzySetMessage=warning
  Scope3 : Scope
  Zero-Order Hold : ZeroOrderHold  SampleTime=Ts
  Out1 : Outport  InitialOutput=0  VectorParamsAs1DForOutWhenUnconnected=off
  wires:
  In1/1 -> Fuzzy Logic Controller/1, Zero-Order Hold/1
  Fuzzy Logic Controller/1 -> Out1/1
  Zero-Order Hold/1 -> Scope3/1

== system Microgrid/Wind/ANFIS Controller with Ruleviewer ==
  In1 : Inport
  Fuzzy Logic Controller : fuzblock/Fuzzy Logic  Controller  FIS='tipper.fis'  OutputSampleNumber=101  DataType=double  FuzzifiedInputs=off  RuleFiringStrengths=off  RuleOutputs=off  AggregatedOutputs=off  SimulateUsing=Interpreted execution  OutOfRangeInputValueMessage=warning  NoRuleFiredMessage=warning  EmptyOutputFuzzySetMessage=warning
  Scope3 : Scope
  Zero-Order Hold : ZeroOrderHold  SampleTime=Ts
  Out1 : Outport  InitialOutput=0  VectorParamsAs1DForOutWhenUnconnected=off
  wires:
  In1/1 -> Fuzzy Logic Controller/1, Zero-Order Hold/1
  Fuzzy Logic Controller/1 -> Out1/1
  Zero-Order Hold/1 -> Scope3/1

== system Microgrid/Wind  Poweer System/ANFIS Controller with Ruleviewer ==
  In1 : Inport
  Fuzzy Logic Controller : fuzblock/Fuzzy Logic  Controller  FIS='tipper.fis'  OutputSampleNumber=101  DataType=double  FuzzifiedInputs=off  RuleFiringStrengths=off  RuleOutputs=off  AggregatedOutputs=off  SimulateUsing=Interpreted execution  OutOfRangeInputValueMessage=warning  NoRuleFiredMessage=warning  EmptyOutputFuzzySetMessage=warning
  Scope3 : Scope
  Zero-Order Hold : ZeroOrderHold  SampleTime=Ts
  Out1 : Outport  InitialOutput=0  VectorParamsAs1DForOutWhenUnconnected=off
  wires:
  In1/1 -> Fuzzy Logic Controller/1, Zero-Order Hold/1
  Fuzzy Logic Controller/1 -> Out1/1
  Zero-Order Hold/1 -> Scope3/1

== system Microgrid/Wind  Poweer System/Pitch_angle-controller1 ==
  wr : Inport
  0-pitch_max : Saturate  UpperLimit=45  LowerLimit=0
  Constant2 : Constant  Value=2
  "Rate Limiter   " : RateLimiter  RisingSlewLimit=2  FallingSlewLimit=-2
  Sum : Sum  Inputs=|+-  SaturateOnIntegerOverflow=on
  genertaor terminal6 : Scope  NumInputPorts=2
  pitch_gain : Gain  Gain=500  SaturateOnIntegerOverflow=on  OutDataTypeStr=Inherit: Same as input  ParamDataTypeStr=Inherit: Same as input
  Pitch_angle : Outport
  wires:
  wr/1 -> Sum/1
  0-pitch_max/1 -> genertaor terminal6/2, "Rate Limiter   "/1
  Constant2/1 -> Sum/2
  Sum/1 -> pitch_gain/1
  pitch_gain/1 -> 0-pitch_max/1
  "Rate Limiter   "/1 -> genertaor terminal6/1, Pitch_angle/1

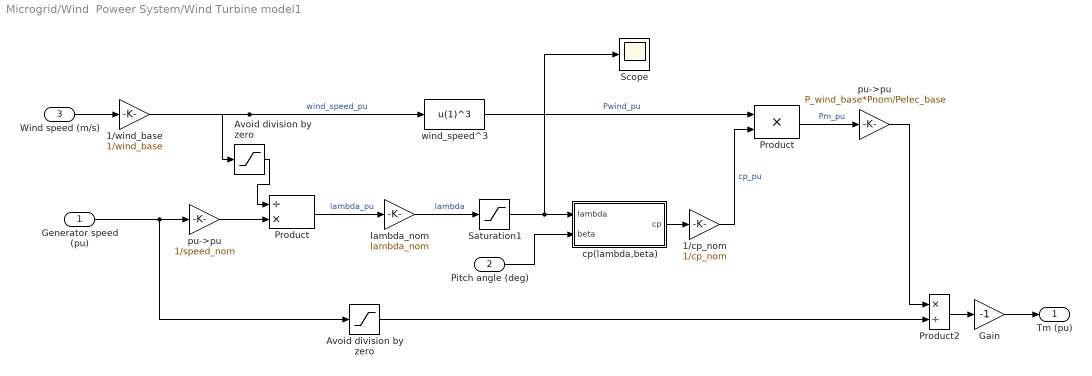
== system Microgrid/Wind  Poweer System/Wind Turbine model1 ==
  Generator speed (pu) : Inport
  Pitch angle (deg) : Inport  Port=2
  Wind speed (m/s) : Inport  Port=3
  1/cp_nom : Gain  Gain=1/cp_nom  SaturateOnIntegerOverflow=on  OutDataTypeStr=Inherit: Same as input  ParamDataTypeStr=Inherit: Same as input
  1/wind_base : Gain  Gain=1/wind_base  SaturateOnIntegerOverflow=on  OutDataTypeStr=Inherit: Same as input  ParamDataTypeStr=Inherit: Same as input
  Avoid division by zero : Saturate  UpperLimit=1e6  LowerLimit=1e-6
  "Avoid division by zero " : Saturate  UpperLimit=1e6  LowerLimit=1e-6
  Gain : Gain  Gain=-1  SaturateOnIntegerOverflow=on  OutDataTypeStr=Inherit: Same as input  ParamDataTypeStr=Inherit: Same as input
  Product : Product  Inputs=/*  SaturateOnIntegerOverflow=on  OutDataTypeStr=Inherit: Same as first input
  "Product " : Product  SaturateOnIntegerOverflow=on  OutDataTypeStr=Inherit: Same as first input
  Product2 : Product  Inputs=*/  InputSameDT=on  SaturateOnIntegerOverflow=on  OutDataTypeStr=Inherit: Same as first input
  Saturation1 : Saturate  UpperLimit=inf  LowerLimit=1e-6
  Scope : Scope
  cp(lambda,beta) : Subsystem
  lambda_nom : Gain  Gain=lambda_nom  SaturateOnIntegerOverflow=on  OutDataTypeStr=Inherit: Same as input  ParamDataTypeStr=Inherit: Same as input
  pu->pu : Gain  Gain=P_wind_base*Pnom/Pelec_base  SaturateOnIntegerOverflow=on  OutDataTypeStr=Inherit: Same as input  ParamDataTypeStr=Inherit: Same as input
  "pu->pu " : Gain  Gain=1/speed_nom  SaturateOnIntegerOverflow=on  OutDataTypeStr=Inherit: Same as input  ParamDataTypeStr=Inherit: Same as input
  wind_speed^3 : Fcn  Expr=u(1)^3
  Tm (pu) : Outport
  wires:
  "pu->pu "/1 -> Product/2
  "Avoid division by zero "/1 -> Product/1
  1/wind_base/1 -> "Avoid division by zero "/1, wind_speed^3/1  "wind_speed_pu"
  Product/1 -> lambda_nom/1  "lambda_pu"
  Saturation1/1 -> Scope/1, cp(lambda,beta)/1(lambda)
  1/cp_nom/1 -> "Product "/2  "cp_pu"
  lambda_nom/1 -> Saturation1/1  "lambda"
  "Product "/1 -> pu->pu/1  "Pm_pu"
  Generator speed (pu)/1 -> "pu->pu "/1, Avoid division by zero/1
  Gain/1 -> Tm (pu)/1
  Wind speed (m/s)/1 -> 1/wind_base/1
  Avoid division by zero/1 -> Product2/2
  Product2/1 -> Gain/1
  wind_speed^3/1 -> "Product "/1  "Pwind_pu"
  cp(lambda,beta)/1(cp) -> 1/cp_nom/1
  pu->pu/1 -> Product2/1
  Pitch angle (deg)/1 -> cp(lambda,beta)/2(beta)

== system Microgrid/Subsystem1/EXCITATION/AC1A ==
  Vref : Inport
  Vt : Inport  Port=2
  It : Inport  Port=3
  Ifd : Inport  Port=4
  Vstab : Inport  Port=5
  AC1A : spsAC1AExcitationSystemLib/AC1A Excitation System  Tr=20e-3  KaTa=[400 0.02]  VAminmax=[-14.5 14.5]  VRminmax=[-5.43 6.03]  KfTf=[0.03 1.0]  TbTc=[0 0]  KeTe=[1.0 0.80]  Ve12=[4.18 3.14]  SeVe12=[0.10 0.03]  Kd=0.38  Kc=0.20  v0=[1 1.4273]  TsBlock=-2
      settings: LibrarySourceBlock=|
      | sps_lib/Electrical Machines/Synchronous Machine Control/AC1A
      | Excitation System
  term3 : Terminator
  Efd : Outport
  wires:
  It/1 -> term3/1
  AC1A/1 -> Efd/1
  Vstab/1 -> AC1A/4
  Ifd/1 -> AC1A/3
  Vt/1 -> AC1A/2
  Vref/1 -> AC1A/1

== system Microgrid/Subsystem1/EXCITATION/AC4A ==
  Vref : Inport
  Vt : Inport  Port=2
  It : Inport  Port=3
  Ifd : Inport  Port=4
  Vstab : Inport  Port=5
  AC4A : spsAC4AExcitationSystemLib/AC4A Excitation System  Tr=20e-3  KaTa=[200 0.015]  VIminmax=[-10 10]  VRminmax=[-4.53 5.64]  TbTc=[10 1.0]  Kc=0  v0=[1,1.42734]  TsBlock=-2
      settings: LibrarySourceBlock=|
      | sps_lib/Electrical Machines/Synchronous Machine Control/AC4A
      | Excitation System
  term3 : Terminator
  Efd : Outport
  wires:
  It/1 -> term3/1
  AC4A/1 -> Efd/1
  Vstab/1 -> AC4A/4
  Ifd/1 -> AC4A/3
  Vt/1 -> AC4A/2
  Vref/1 -> AC4A/1

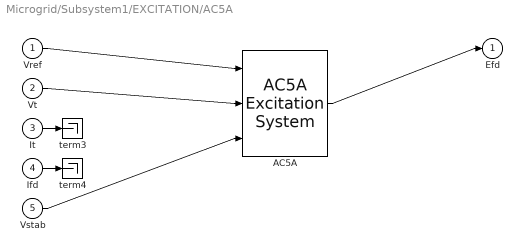
== system Microgrid/Subsystem1/EXCITATION/AC5A ==
  Vref : Inport
  Vt : Inport  Port=2
  It : Inport  Port=3
  Ifd : Inport  Port=4
  Vstab : Inport  Port=5
  AC5A : spsAC5AExcitationSystemLib/AC5A Excitation System  Tr=20e-3  KaTa=[100 0.02]  VRminmax=[-7.3 7.3]  KfTf=[0.03 1 0 0]  KeTe=[1.0 0.02]  Efd12=[5.6 0.75*5.6]  SeEfd12=[0.86 0.5]  v0=[1,1.42734]  TsBlock=-2
      settings: LibrarySourceBlock=|
      | sps_lib/Electrical Machines/Synchronous Machine Control/AC5A
      | Excitation System
  term3 : Terminator
  term4 : Terminator
  Efd : Outport
  wires:
  Ifd/1 -> term4/1
  It/1 -> term3/1
  AC5A/1 -> Efd/1
  Vstab/1 -> AC5A/3
  Vt/1 -> AC5A/2
  Vref/1 -> AC5A/1

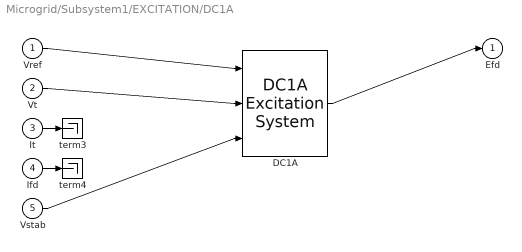
== system Microgrid/Subsystem1/EXCITATION/DC1A ==
  Vref : Inport
  Vt : Inport  Port=2
  It : Inport  Port=3
  Ifd : Inport  Port=4
  Vstab : Inport  Port=5
  DC1A : spsDC1AExcitationSystemLib/DC1A Excitation System  Tr=20e-3  KaTa=[46 0.06]  VRminmax=[-0.9 1.0]  KfTf=[0.05 1.5]  TbTc=[0 0]  KeTe=[0.05 0.46]  Efd12=[3.1 2.3]  SeEfd12=[0.33 0.10]  v0=[1,1.42734]  TsBlock=-2
      settings: LibrarySourceBlock=|
      | sps_lib/Electrical Machines/Synchronous Machine Control/DC1A
      | Excitation System
  term3 : Terminator
  term4 : Terminator
  Efd : Outport
  wires:
  Ifd/1 -> term4/1
  It/1 -> term3/1
  DC1A/1 -> Efd/1
  Vstab/1 -> DC1A/3
  Vt/1 -> DC1A/2
  Vref/1 -> DC1A/1

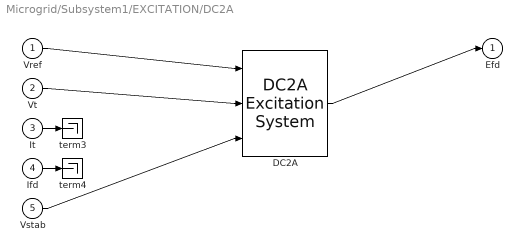
== system Microgrid/Subsystem1/EXCITATION/DC2A ==
  Vref : Inport
  Vt : Inport  Port=2
  It : Inport  Port=3
  Ifd : Inport  Port=4
  Vstab : Inport  Port=5
  DC2A : spsDC2AExcitationSystemLib/DC2A Excitation System  Tr=20e-3  KaTa=[46 0.06]  VRminmax=[-4.9 4.95]  KfTf=[0.05 1.5]  TbTc=[0 0]  KeTe=[0.05 0.46]  Efd12=[3.05 2.29]  SeEfd12=[0.279 0.117]  v0=[1,1.42734]  TsBlock=-2
      settings: LibrarySourceBlock=|
      | sps_lib/Electrical Machines/Synchronous Machine Control/DC2A
      | Excitation System
  term3 : Terminator
  term4 : Terminator
  Efd : Outport
  wires:
  Ifd/1 -> term4/1
  It/1 -> term3/1
  DC2A/1 -> Efd/1
  Vstab/1 -> DC2A/3
  Vt/1 -> DC2A/2
  Vref/1 -> DC2A/1

== system Microgrid/Subsystem1/EXCITATION/ST1A ==
  Vref : Inport
  Vt : Inport  Port=2
  It : Inport  Port=3
  Ifd : Inport  Port=4
  Vstab : Inport  Port=5
  ST1A : spsST1AExcitationSystemLib/ST1A Excitation System  Tr=20e-3  KaTa=[210 0.001]  VIminmax=[-999 999]  VAminmax=[-999 999]  VRminmax=[-6.0 6.43]  KfTf=[0.001 1]  TbTc=[0 0 0 0]  KLR=1  ILR=2  Kc=0.038  v0=[1,1.42734]  TsBlock=-2
      settings: LibrarySourceBlock=|
      | sps_lib/Electrical Machines/Synchronous Machine Control/ST1A
      | Excitation System
  term3 : Terminator
  Efd : Outport
  wires:
  It/1 -> term3/1
  ST1A/1 -> Efd/1
  Vstab/1 -> ST1A/4
  Ifd/1 -> ST1A/3
  Vt/1 -> ST1A/2
  Vref/1 -> ST1A/1

== system Microgrid/Wind  Poweer System/Wind Turbine model1/cp(lambda,beta) ==
  lambda : Inport
  beta : Inport  Port=2
  Fcn : Fcn  Expr=1/(1/(u[1]+0.08*u[2])-0.035/(u[2]^3+1))
  Fcn1 : Fcn  Expr=sin(u(1)*exp(2.3*(-u(2))))
  Mux : Mux  Inputs=2
  Mux1 : Mux  Inputs=3
  cp : Outport
  wires:
  Mux/1 -> Fcn/1
  beta/1 -> Mux/2, Mux1/3
  Mux1/1 -> Fcn1/1
  lambda/1 -> Mux/1, Mux1/1
  Fcn1/1 -> cp/1
  Fcn/1 -> Mux1/2  "lambda_i"
